simulink model "RetinaGuard_SimEvents_Day1_Verified"  (R2026a)
settings: Solver=VariableStepAuto  StopTime=480
settings Model: Creator=NITIN  LastModifiedBy=NITIN

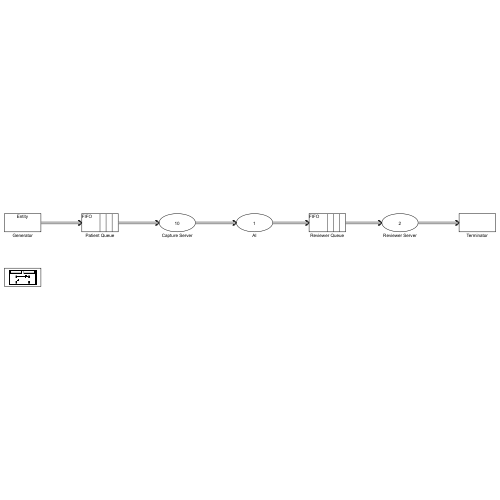
[thumbnail: Simulink's stored preview of the top-level diagram]
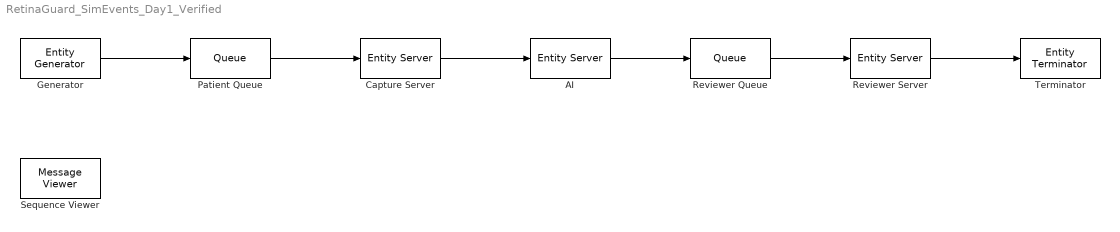
== system RetinaGuard_SimEvents_Day1_Verified ==
  AI : EntityServer  InputPortMessageModes=m  OutputPortMessageModes=m  Capacity=1  ServiceTimeValue=3
  Capture Server : EntityServer  InputPortMessageModes=m  OutputPortMessageModes=m  Capacity=10  ServiceTimeValue=5
  Generator : EntityGenerator  OutputPortMessageModes=m  EntityType=Structured  EntityTypeName=Entity
  Patient Queue : Queue  InputPortMessageModes=m  OutputPortMessageModes=m  Capacity=500
  Reviewer Queue : Queue  InputPortMessageModes=m  OutputPortMessageModes=m  Capacity=500
  Reviewer Server : EntityServer  InputPortMessageModes=m  OutputPortMessageModes=m  Capacity=2  ServiceTimeValue=3
  Sequence Viewer : MessageViewer  History=1000  SavedRootId=#
  Terminator : EntityTerminator  InputPortMessageModes=m
  wires:
  Generator/1 -> Patient Queue/1
  Patient Queue/1 -> Capture Server/1
  Capture Server/1 -> AI/1
  AI/1 -> Reviewer Queue/1
  Reviewer Queue/1 -> Reviewer Server/1
  Reviewer Server/1 -> Terminator/1
